simulink library "INT_CoVM_TrqDesCoord"  (R2016b)
settings: Solver=VariableStepAuto  StartTime=0.0  StopTime=10.0  RelTol=1e-3
settings Model: Creator=bianxuyin  LastModifiedBy=bianxuyin

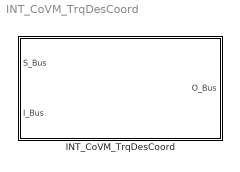
== system INT_CoVM_TrqDesCoord ==
  INT_CoVM_TrqDesCoord : Subsystem

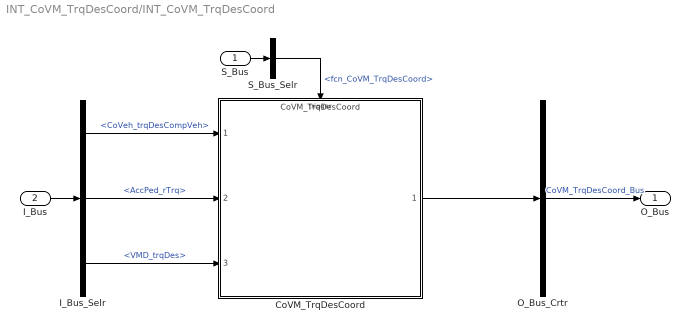
== system INT_CoVM_TrqDesCoord/INT_CoVM_TrqDesCoord ==
  S_Bus : Inport
  I_Bus : Inport  Port=2
  CoVM_TrqDesCoord : ModelReference  ModelNameDialog=CoVM_TrqDesCoord  SimulationMode=Normal  ModelReferenceVersion=1.4  TriggerPortName=function  TriggerPortTriggerType=function-call  TriggerPortStatesWhenEnabling=held
  I_Bus_Selr : BusSelector  OutputSignals=CoVeh_trqDesCompVeh,AccPed_rTrq,VMD_trqDes
  O_Bus_Crtr : BusCreator  Inputs=1
  S_Bus_Selr : BusSelector  OutputSignals=fcn_CoVM_TrqDesCoord
  O_Bus : Outport
  wires:
  S_Bus_Selr/1 -> CoVM_TrqDesCoord/Trigger  "<fcn_CoVM_TrqDesCoord>"
  S_Bus/1 -> S_Bus_Selr/1
  I_Bus/1 -> I_Bus_Selr/1
  I_Bus_Selr/1 -> CoVM_TrqDesCoord/1  "<CoVeh_trqDesCompVeh>"
  I_Bus_Selr/2 -> CoVM_TrqDesCoord/2  "<AccPed_rTrq>"
  I_Bus_Selr/3 -> CoVM_TrqDesCoord/3  "<VMD_trqDes>"
  O_Bus_Crtr/1 -> O_Bus/1  "CoVM_TrqDesCoord_Bus"
  CoVM_TrqDesCoord/1 -> O_Bus_Crtr/1
